simulink model "TASK5_initial_poles"  (R2023b)
settings: Solver=VariableStepAuto  StartTime=0.0  StopTime=10  MaxStep=0.01  RelTol=1e-3  EnableMultiTasking=on
values from neighbouring files (symbols this model uses):
  b = 0.2    [TASK0_main_code.m]
  dphi0 = 0.1    [TASK0_main_code.m]
  dx0 = 0.01    [TASK0_main_code.m]
  g = 9.81    [TASK0_main_code.m]
  J_s = 1/3*m*l^2    (= 4.99725166667)    [TASK0_main_code.m]
  K = place(A_lin, B_lin, p)    [TASK0_main_code.m]
  l = 3.11    [TASK0_main_code.m]
  m = 1.55    [TASK0_main_code.m]
  M = 7.87    [TASK0_main_code.m]
  phi0 = 0.05    [TASK0_main_code.m]
  x0 = -0.01    [TASK0_main_code.m]
libraries: dspinverses x1
settings Model: Creator=iklod_000  LastModifiedBy=piri
settings SolverCC: AlgebraicLoopSolver=TrustRegion
settings DataIOCC: ReturnWorkspaceOutputs=off
settings OptimizationCC: LifeSpan=inf
settings DebuggingCC: UnconnectedInputMsg=warning  UnconnectedOutputMsg=warning  UnconnectedLineMsg=warning  SFUnexpectedBacktrackingDiag=warning  SFNoUnconditionalDefaultTransitionDiag=warning  ArithmeticOperatorsInVariantConditions=warning
settings ModelReferenceCC: EnableRefExpFcnMdlSchedulingChecks=on
settings SFSimCC: SimUseLocalCustomCode=off  CustomCodeUndefinedFunction=UseInterfaceOnly
settings RTWCC: RTWUseLocalCustomCode=off
settings CodeAppCC: StateflowObjectComments=on
settings GRTTargetCC: TargetLangStandard=C89/C90 (ANSI)
settings ConfigComp: CovMetricSettings=dw  CovSaveCumulativeToWorkspaceVar=on  CovSaveSingleToWorkspaceVar=on  CovExternalEMLEnable=off

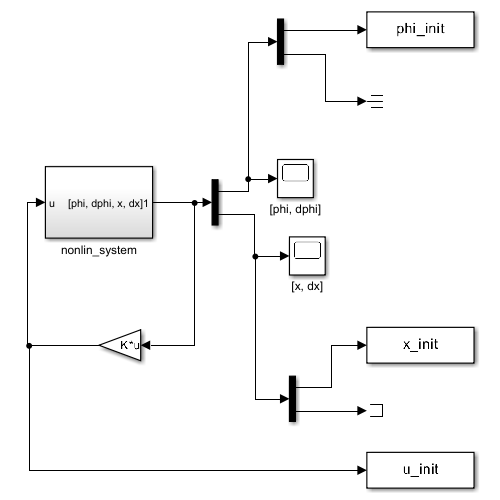
[thumbnail: Simulink's stored preview of the top-level diagram]
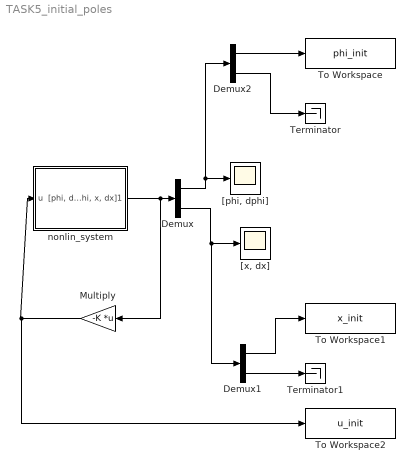
== system TASK5_initial_poles ==
  Demux : Demux  Outputs=2
  Demux1 : Demux  Outputs=2
  Demux2 : Demux  Outputs=2
  Multiply : Gain  Gain=-K  Multiplication=Matrix(K*u)
  Terminator : Terminator
  Terminator1 : Terminator
  To Workspace : ToWorkspace  VariableName=phi_init  SaveFormat=Timeseries  SampleTime=-1
  To Workspace1 : ToWorkspace  VariableName=x_init  SaveFormat=Timeseries  SampleTime=-1
  To Workspace2 : ToWorkspace  VariableName=u_init  SaveFormat=Timeseries  SampleTime=-1
  "[phi, dphi] " : Scope
  "[x, dx]" : Scope
  nonlin_system : Subsystem
  wires:
  nonlin_system/1("[phi, dphi, x, dx]1") -> Multiply/1, Demux/1
  Demux/1 -> Demux2/1, "[phi, dphi] "/1
  Demux/2 -> Demux1/1, "[x, dx]"/1
  Multiply/1 -> To Workspace2/1, nonlin_system/1(u)
  Demux1/2 -> Terminator1/1
  Demux1/1 -> To Workspace1/1
  Demux2/1 -> To Workspace/1
  Demux2/2 -> Terminator/1

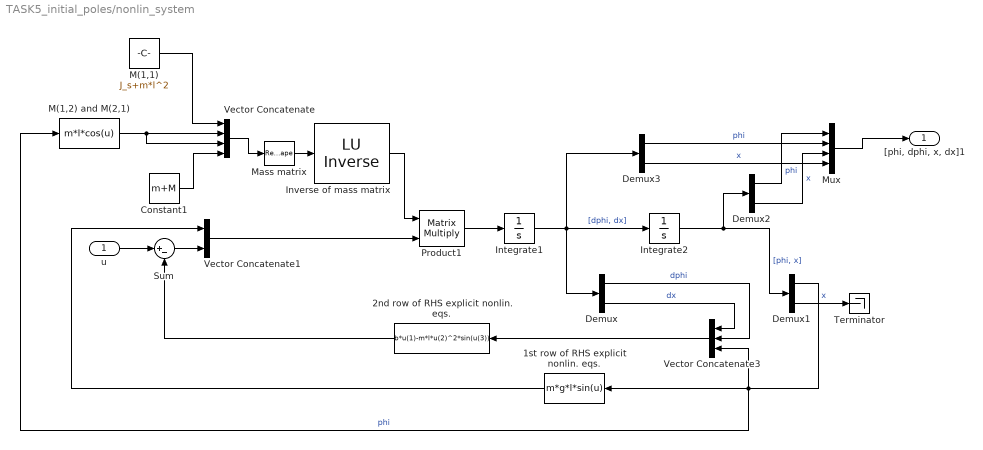
== system TASK5_initial_poles/nonlin_system ==
  u : Inport
  1st row of RHS explicit nonlin. eqs. : Fcn  Expr=m*g*l*sin(u)
  2nd row of RHS explicit nonlin. eqs. : Fcn  Expr=b*u(1)-m*l*u(2)^2*sin(u(3))
  Constant1 : Constant  Value=m+M
  Demux{,1..3} (4 alike) : Demux  Outputs=2
  Integrate1 : Integrator  InitialCondition=[dphi0; dx0]
  Integrate2 : Integrator  InitialCondition=[phi0; x0]
  Inverse of mass matrix : dspinverses/ LU Inverse
  M(1,1) : Constant  Value=J_s+m*l^2
  M(1,2) and M(2,1) : Fcn  Expr=m*l*cos(u)
  Mass matrix : Reshape  OutputDimensionality=Customize  OutputDimensions=[2,2]
  Mux : Mux
  Product1 : Product  Multiplication=Matrix(*)
  Sum : Sum  Inputs=|+-
  Terminator : Terminator
  Vector Concatenate : Concatenate  NumInputs=4
  Vector Concatenate1 : Concatenate
  Vector Concatenate3 : Concatenate  NumInputs=3
  "[phi, dphi, x, dx]1" : Outport
  wires:
  Mass matrix/1 -> Inverse of mass matrix/1
  u/1 -> Sum/1
  Constant1/1 -> Vector Concatenate/4
  Inverse of mass matrix/1 -> Product1/1
  Vector Concatenate3/1 -> 2nd row of RHS explicit nonlin. eqs./1
  Vector Concatenate1/1 -> Product1/2
  1st row of RHS explicit nonlin. eqs./1 -> Vector Concatenate1/1
  Sum/1 -> Vector Concatenate1/2
  2nd row of RHS explicit nonlin. eqs./1 -> Sum/2
  Vector Concatenate/1 -> Mass matrix/1
  M(1,1)/1 -> Vector Concatenate/1
  M(1,2) and M(2,1)/1 -> Vector Concatenate/3, Vector Concatenate/2
  Product1/1 -> Integrate1/1
  Integrate1/1 -> Demux3/1, Demux/1, Integrate2/1  "[dphi, dx]"
  Integrate2/1 -> Demux2/1, Demux1/1  "[phi, x]"
  Demux/2 -> Vector Concatenate3/1  "dx"
  Demux/1 -> Vector Concatenate3/2  "dphi"
  Demux1/1 -> 1st row of RHS explicit nonlin. eqs./1, M(1,2) and M(2,1)/1, Vector Concatenate3/3  "phi"
  Demux2/1 -> Mux/1  "phi"
  Mux/1 -> "[phi, dphi, x, dx]1"/1
  Demux3/1 -> Mux/2  "phi"
  Demux2/2 -> Mux/3  "x"
  Demux3/2 -> Mux/4  "x"
  Demux1/2 -> Terminator/1  "x"
